simulink model "pfc_desktop"  (R2024b)
settings: configuration reference "CONFI" (kept outside this file)
InitFcn:
  | fidelity_pfc_vals;
  | Fc=66e3;
values from neighbouring files (symbols this model uses):
  Gs = 2e-2    (= 0.02)    [fidelity_pfc_vals.m]
  s = 1    [fidelity_pfc_vals.m]
  stateSpaceParameters_1 =     [stateSpaceParameters.mat]
  t_ss = tsw/30    (= 5.12820512821e-07)    [fidelity_pfc_vals.m]
  tsw = 1/(fsw*1e3)    (= 1.53846153846e-05)    [fidelity_pfc_vals.m]
undefined symbols (not defined in the file or in its folder): a, b, c, DiscIntNeverNeededParam, Down, Up
libraries: fl_lib x40, nesl_utility x37, ee_lib x11, hdlsllib x7, dspsrcs4 x6, eePwmGenerator x3, hdlssclib x2, spsTriangleGeneratorLib x1, simulink x1
(part 3 of 3)

== system pfc_desktop/simscape_system/3Bridges/Simscape/Subsystem5 ==
  g : Inport
  "MOSFET (Ideal, Switching)" : ee_lib/Semiconductors & Converters/MOSFET (Ideal, Switching)  port_option=ee.enum.controlport.ps  Rds=0.01 Ohm  Goff=1e-6 1/Ohm  Vth=2 V  diode_param=ee.enum.semiconductors.protectionDiode.nodynamics  diode_Vf=0.8 V  diode_Ron=0.001 Ohm  diode_Goff=1e-5 1/Ohm  diode_C=50e-9 F  diode_iRM=-235 A  diode_iF=300 A  diode_idot=-50 A/us  diode_trr_param=ee.enum.converters.diodeReverseParam.trr_factor  diode_trr_factor=3  diode_trr=15 us  diode_Qrr=1500 s*uA  ids_specify=off  ids_priority=None  ids=0 A  ids_nominal_specify=off  ids_nominal_value=1  ids_nominal_unit=A  vds_specify=off  vds_priority=None  vds=0 V  vds_nominal_specify=off  vds_nominal_value=1  vds_nominal_unit=V  vgs_specify=off  vgs_priority=None  vgs=0 V  vgs_nominal_specify=off  vgs_nominal_value=1  vgs_nominal_unit=V  thermal_loss_option=ee.enum.converters.thermalLossOption.constantvalues  Von_data=[0, 1.8, 3.2, 6, 10, 16; 0, 2, 5.5, 9.5, 15, 25] V  Tj=[298.15, 448.15] K  Iout_data=[0, 20, 40, 60, 80, 100] A  Eon_data=[0, 55.04, 124.57, 235.53, 362.12; 0, 71.25, 161.25, 304.88, 468.75] * 1e-6 J  Eoff_data=[0, 18, 30, 56.1, 76.5; 0, 22.5, 37.5, 70.13, 95.63] * 1e-6 J  Eon_data_3D=[zeros(2, 5, 3)] J  Eoff_data_3D=[zeros(2, 5, 3)] J  Tj_loss=[298.15, 448.15] K  Iout_data_loss=[0, 10, 20, 30, 40] A  tabulateWithVds=false  Vds_loss=[0, 150, 300] V  Eon_scalar=22.86e-3 J  Eoff_scalar=17.14e-3 J  Voff=300 V  Iout_scalar=600 A  useCurrentFromPreviousCycle=false  useVoltageFromPreviousCycle=false  diodeModelType=ee.enum.converters.diodeModelType.pwl  diodeTableType=ee.enum.diode.tableType.IfMat  diode_ReverseIVType=ee.enum.diode.diodeReverseIV.constant  diode_IfMat=[.07, .12, .19, 1.75, 4.24, 7.32, 11.2; .16, .3, .72, 2.14, 4.02, 6.35, 9.12] A  diode_VfMat=[.9, 1.15, 1.25, 1.5, 1.75, 2.17, 2.6, 2.85; .58, .68, .75, 1.1, 1.38, 1.77, 2.27, 2.7] V  diode_TjVec=[25, 125] degC  diode_VfVec=[.5, .7, .9, 1.3, 1.7, 2.1, 2.5] V  diode_IfVec=[.1, .2, .5, 1, 2, 4, 7, 10] A  diode_IrMat=[1e-06, 2e-06, 5e-06, 1e-05, 2.5e-05, 5e-05, .0001; 2e-06, 5e-06, 1e-05, 4e-05, 8e-05, .0002, .0005] A  diode_VrMat=[10, 100, 200, 250, 300, 325, 350; 10, 70, 160, 220, 270, 300, 320] V  diode_VrVec=[10, 20, 40, 50, 70, 80, 100] V  diode_IrVec=[1e-06, 2e-06, 5e-06, 1e-05, 2e-05, 5e-05, .0001] A  diode_Vr=-600 V  diode_Ls=150 nH  diode_Erec=0.03 J  diode_rec_loss_model=ee.enum.diode.reverseRecoveryModel.fixed  diode_ErecVal=0 J  diode_scaleWithIandV=true  diode_ErecMat=zeros(2, 3) J  diode_TjrecVec=[298.15, 398.15] K  diode_IfrecVec=[.1, 1, 10] A  diode_IrecVal=10 A  diode_VrecVal=10 V  diode_tFilter=1 / 1000 / 100 s  separateThermalPortForDiode=false  thermal_network_parameterization=ee.enum.thermalNetworkTopology.external  Rth=[.03, .2] K/W  Rth_Cauer=[.03, .1, .2] K/W  Rth_Foster=[.08, .14, .22, .16] K/W  thermal_mass_parameterization=ee.enum.thermalNetwork.timeconstant  thermal_mass=[3, 25] J/K  thermal_mass_Cauer=[3, 10, 25] J/K  thermal_mass_Foster=[.001, .005, .05, .5] J/K  thermal_time_constant=[.1, 5] s  thermal_time_constant_Cauer=[.1, 1, 5] s  thermal_time_constant_Foster=[7e-05, .0007, .01, .08] s  thermal_mass_initial_temperatures=[25, 25] degC  thermal_mass_initial_temperatures_Cauer=[25, 25, 25] degC  junction_thermal_mass=0.1 J/K  Tvec_initial_Foster=[25, 25, 25, 25] degC  RthDiode=[.03, .2] K/W  RthCauerDiode=[.03, .1, .2] K/W  RthFosterDiode=[.03, .2] K/W  thermalMassDiode=[3, 25] J/K  thermalMassCauerDiode=[3, 10, 25] J/K  thermalMassFosterDiode=[33, 50] J/K  thermalTauDiode=[.1, 5] s  thermalTauCauerDiode=[.1, 1, 5] s  thermalTauFosterDiode=[1, 10] s  thermalMassInitTempDiode=[25, 25] degC  thermalMassInitTempCauerDiode=[25, 25, 25] degC  junctionthermalMassDiode=0.1 J/K  TVecInitialFosterDiode=[25, 25, 25, 25] degC  no_thermal_network=0  mosfet_junction_temperature_specify=off  mosfet_junction_temperature_priority=None  mosfet_junction_temperature=25 degC  mosfet_junction_temperature_nominal_specify=off  mosfet_junction_temperature_nominal_value=1  mosfet_junction_temperature_nominal_unit=degC  diode_junction_temperature_specify=off  diode_junction_temperature_priority=None  diode_junction_temperature=25 degC  diode_junction_temperature_nominal_specify=off  diode_junction_temperature_nominal_value=1  diode_junction_temperature_nominal_unit=degC  Qj_specify=off  Qj_priority=None  Qj=0 W  Qj_nominal_specify=off  Qj_nominal_value=1  Qj_nominal_unit=W  accumulatedSwitchingLosses_specify=off  accumulatedSwitchingLosses_priority=None  accumulatedSwitchingLosses=0 J
  Simulink-PS Converter : nesl_utility/Simulink-PS Converter  PhysicalDomain=network_engine_domain  SubClassName=ps_input  LeftPortType=input  RightPortType=output  PseudoPeriodic=off  Frequencies=[]  NoiseDistribution=none  NoiseParameters=[]  Unit=1  AffineConversion=off  FilteringAndDerivatives=provide  SimscapeFilterOrder=1  InputFilterTimeConstant=0.001  UdotUserProvided=0
  d : PMIOPort  Side=Left
  s : PMIOPort  Port=2  Side=Right
  wires:
  g/1 -> Simulink-PS Converter/1
  connections:
  "MOSFET (Ideal, Switching)"/RConn1 -- d/RConn1
  "MOSFET (Ideal, Switching)"/RConn2 -- s/RConn1
  Simulink-PS Converter/RConn1 -- "MOSFET (Ideal, Switching)"/LConn1

== system pfc_desktop/simscape_system1/HDL Subsystem/HDL Algorithm/Output ==
  In1 : Inport
  State : Inport  Port=2
  Sel : Inport  Port=3  LockScale=on
  Bias : Terminator
  Mux : Mux  Inputs=2
  Output Update : hdlssclib/NFPSparseConstMultiply  MatrixSource=Dialog  constMatrix=single([stateSpaceParameters_1.Cd stateSpaceParameters_1.Dd])  MatrixType=single  MatrixSize=[1 1]  ColumnIndices=[1]  RowIndices=[1]  PropDataType=single  defWL=48
  Out1 : Outport  VectorParamsAs1DForOutWhenUnconnected=off
  wires:
  State/1 -> Mux/1
  Mux/1 -> Output Update/1
  In1/1 -> Mux/2
  Sel/1 -> Bias/1, Output Update/2
  Output Update/1 -> Out1/1

== system pfc_desktop/simscape_system1/HDL Subsystem/HDL Algorithm/State Update ==
  In1 : Inport
  State : Inport  Port=2
  Sel : Inport  Port=3  LockScale=on
  Bias : Terminator
  Mux : Mux  Inputs=2
  State Update : hdlssclib/NFPSparseConstMultiply  MatrixSource=Dialog  constMatrix=single([stateSpaceParameters_1.Ad stateSpaceParameters_1.Bd])  MatrixType=single  MatrixSize=[1 1]  ColumnIndices=[1]  RowIndices=[1]  PropDataType=single  defWL=43
  State Out : Outport  VectorParamsAs1DForOutWhenUnconnected=off
  wires:
  State/1 -> Mux/1
  In1/1 -> Mux/2
  Mux/1 -> State Update/1
  Sel/1 -> Bias/1, State Update/2
  State Update/1 -> State Out/1

== system pfc_desktop/simscape_system/3Bridges/Linear_FET/MOSFET/Controller ==
  vs : Inport
  is : Inport  Port=2
  G : Inport  Port=3
  Constant : Constant  Value=-.7  SampleTime=-1
  Discrete-Time Integrator : DiscreteIntegrator  IntegratorMethod=Accumulation: Forward Euler  gainval=1/s  SampleTime=-1  OutDataTypeStr=Inherit: Inherit via back propagation  ICPrevOutput=DiscIntNeverNeededParam  ICPrevScaledInput=DiscIntNeverNeededParam
  Equal : RelationalOperator  OutDataTypeStr=boolean  RndMeth=Simplest  InputSameDT=off
  Gain : Gain  Gain=10
  Gain3 : Gain  Gain=Gs  OutDataTypeStr=Inherit: Inherit via back propagation
  Multiply-Add : hdlsllib/HDL Operations/Multiply-Add  Function=c+(a.*b)  datatype=Inherit: Inherit via internal rule  DoSatur=off  FMA=off
  OR : Logic  Operator=OR  IconShape=distinctive  AllPortsSameDT=off  OutDataTypeStr=boolean
  Subtract : Sum  Inputs=+-
  Subtract1 : Sum  Inputs=+-
  Unary Minus : UnaryMinus
  ic : Outport
  wires:
  Multiply-Add/1 -> Subtract/1
  G/1 -> OR/1
  Unary Minus/1 -> Subtract1/1  "on"
  is/1 -> Unary Minus/1
  Discrete-Time Integrator/1 -> ic/1, Subtract/2  "ic"
  Subtract/1 -> Discrete-Time Integrator/1
  vs/1 -> Equal/2, Gain3/1
  Equal/1 -> Gain/1
  Gain/1 -> OR/2
  Constant/1 -> Equal/1
  Gain3/1 -> Subtract1/2, Multiply-Add/3
  Subtract1/1 -> Multiply-Add/1
  OR/1 -> Multiply-Add/2

== system pfc_desktop/simscape_system/3Bridges/Linear_FET/MOSFET1/Controller ==
  vs : Inport
  is : Inport  Port=2
  G : Inport  Port=3
  Constant : Constant  Value=-.7  SampleTime=-1
  Discrete-Time Integrator : DiscreteIntegrator  IntegratorMethod=Accumulation: Forward Euler  gainval=1/s  SampleTime=-1  OutDataTypeStr=Inherit: Inherit via back propagation  ICPrevOutput=DiscIntNeverNeededParam  ICPrevScaledInput=DiscIntNeverNeededParam
  Equal : RelationalOperator  OutDataTypeStr=boolean  RndMeth=Simplest  InputSameDT=off
  Gain : Gain  Gain=10
  Gain3 : Gain  Gain=Gs  OutDataTypeStr=Inherit: Inherit via back propagation
  Multiply-Add : hdlsllib/HDL Operations/Multiply-Add  Function=c+(a.*b)  datatype=Inherit: Inherit via internal rule  DoSatur=off  FMA=off
  OR : Logic  Operator=OR  IconShape=distinctive  AllPortsSameDT=off  OutDataTypeStr=boolean
  Subtract : Sum  Inputs=+-
  Subtract1 : Sum  Inputs=+-
  Unary Minus : UnaryMinus
  ic : Outport
  wires:
  OR/1 -> Multiply-Add/2
  Subtract1/1 -> Multiply-Add/1
  Gain3/1 -> Multiply-Add/3, Subtract1/2
  Constant/1 -> Equal/1
  Gain/1 -> OR/2
  Equal/1 -> Gain/1
  vs/1 -> Gain3/1, Equal/2
  Subtract/1 -> Discrete-Time Integrator/1
  Discrete-Time Integrator/1 -> Subtract/2, ic/1  "ic"
  is/1 -> Unary Minus/1
  Unary Minus/1 -> Subtract1/1  "on"
  G/1 -> OR/1
  Multiply-Add/1 -> Subtract/1

== system pfc_desktop/simscape_system/3Bridges/Linear_FET/MOSFET2/Controller ==
  vs : Inport
  is : Inport  Port=2
  G : Inport  Port=3
  Constant : Constant  Value=-.7  SampleTime=-1
  Discrete-Time Integrator : DiscreteIntegrator  IntegratorMethod=Accumulation: Forward Euler  gainval=1/s  SampleTime=-1  OutDataTypeStr=Inherit: Inherit via back propagation  ICPrevOutput=DiscIntNeverNeededParam  ICPrevScaledInput=DiscIntNeverNeededParam
  Equal : RelationalOperator  OutDataTypeStr=boolean  RndMeth=Simplest  InputSameDT=off
  Gain : Gain  Gain=10
  Gain3 : Gain  Gain=Gs  OutDataTypeStr=Inherit: Inherit via back propagation
  Multiply-Add : hdlsllib/HDL Operations/Multiply-Add  Function=c+(a.*b)  datatype=Inherit: Inherit via internal rule  DoSatur=off  FMA=off
  OR : Logic  Operator=OR  IconShape=distinctive  AllPortsSameDT=off  OutDataTypeStr=boolean
  Subtract : Sum  Inputs=+-
  Subtract1 : Sum  Inputs=+-
  Unary Minus : UnaryMinus
  ic : Outport
  wires:
  Multiply-Add/1 -> Subtract/1
  G/1 -> OR/1
  Unary Minus/1 -> Subtract1/1  "on"
  is/1 -> Unary Minus/1
  Discrete-Time Integrator/1 -> ic/1, Subtract/2  "ic"
  Subtract/1 -> Discrete-Time Integrator/1
  vs/1 -> Equal/2, Gain3/1
  Equal/1 -> Gain/1
  Gain/1 -> OR/2
  Constant/1 -> Equal/1
  Gain3/1 -> Subtract1/2, Multiply-Add/3
  Subtract1/1 -> Multiply-Add/1
  OR/1 -> Multiply-Add/2

== system pfc_desktop/simscape_system/3Bridges/Linear_FET/MOSFET3/Controller ==
  vs : Inport
  is : Inport  Port=2
  G : Inport  Port=3
  Constant : Constant  Value=-.7  SampleTime=-1
  Discrete-Time Integrator : DiscreteIntegrator  IntegratorMethod=Accumulation: Forward Euler  gainval=1/s  SampleTime=-1  OutDataTypeStr=Inherit: Inherit via back propagation  ICPrevOutput=DiscIntNeverNeededParam  ICPrevScaledInput=DiscIntNeverNeededParam
  Equal : RelationalOperator  OutDataTypeStr=boolean  RndMeth=Simplest  InputSameDT=off
  Gain : Gain  Gain=10
  Gain3 : Gain  Gain=Gs  OutDataTypeStr=Inherit: Inherit via back propagation
  Multiply-Add : hdlsllib/HDL Operations/Multiply-Add  Function=c+(a.*b)  datatype=Inherit: Inherit via internal rule  DoSatur=off  FMA=off
  OR : Logic  Operator=OR  IconShape=distinctive  AllPortsSameDT=off  OutDataTypeStr=boolean
  Subtract : Sum  Inputs=+-
  Subtract1 : Sum  Inputs=+-
  Unary Minus : UnaryMinus
  ic : Outport
  wires:
  OR/1 -> Multiply-Add/2
  Subtract1/1 -> Multiply-Add/1
  Gain3/1 -> Multiply-Add/3, Subtract1/2
  Constant/1 -> Equal/1
  Gain/1 -> OR/2
  Equal/1 -> Gain/1
  vs/1 -> Gain3/1, Equal/2
  Subtract/1 -> Discrete-Time Integrator/1
  Discrete-Time Integrator/1 -> Subtract/2, ic/1  "ic"
  is/1 -> Unary Minus/1
  Unary Minus/1 -> Subtract1/1  "on"
  G/1 -> OR/1
  Multiply-Add/1 -> Subtract/1

== system pfc_desktop/simscape_system/3Bridges/Linear_FET/MOSFET4/Controller ==
  vs : Inport
  is : Inport  Port=2
  G : Inport  Port=3
  Constant : Constant  Value=-.7  SampleTime=-1
  Discrete-Time Integrator : DiscreteIntegrator  IntegratorMethod=Accumulation: Forward Euler  gainval=1/s  SampleTime=-1  OutDataTypeStr=Inherit: Inherit via back propagation  ICPrevOutput=DiscIntNeverNeededParam  ICPrevScaledInput=DiscIntNeverNeededParam
  Equal : RelationalOperator  OutDataTypeStr=boolean  RndMeth=Simplest  InputSameDT=off
  Gain : Gain  Gain=10
  Gain3 : Gain  Gain=Gs  OutDataTypeStr=Inherit: Inherit via back propagation
  Multiply-Add : hdlsllib/HDL Operations/Multiply-Add  Function=c+(a.*b)  datatype=Inherit: Inherit via internal rule  DoSatur=off  FMA=off
  OR : Logic  Operator=OR  IconShape=distinctive  AllPortsSameDT=off  OutDataTypeStr=boolean
  Subtract : Sum  Inputs=+-
  Subtract1 : Sum  Inputs=+-
  Unary Minus : UnaryMinus
  ic : Outport
  wires:
  Multiply-Add/1 -> Subtract/1
  G/1 -> OR/1
  Unary Minus/1 -> Subtract1/1  "on"
  is/1 -> Unary Minus/1
  Discrete-Time Integrator/1 -> ic/1, Subtract/2  "ic"
  Subtract/1 -> Discrete-Time Integrator/1
  vs/1 -> Equal/2, Gain3/1
  Equal/1 -> Gain/1
  Gain/1 -> OR/2
  Constant/1 -> Equal/1
  Gain3/1 -> Subtract1/2, Multiply-Add/3
  Subtract1/1 -> Multiply-Add/1
  OR/1 -> Multiply-Add/2

== system pfc_desktop/simscape_system/3Bridges/Linear_FET/MOSFET5/Controller ==
  vs : Inport
  is : Inport  Port=2
  G : Inport  Port=3
  Constant : Constant  Value=-.7  SampleTime=-1
  Discrete-Time Integrator : DiscreteIntegrator  IntegratorMethod=Accumulation: Forward Euler  gainval=1/s  SampleTime=-1  OutDataTypeStr=Inherit: Inherit via back propagation  ICPrevOutput=DiscIntNeverNeededParam  ICPrevScaledInput=DiscIntNeverNeededParam
  Equal : RelationalOperator  OutDataTypeStr=boolean  RndMeth=Simplest  InputSameDT=off
  Gain : Gain  Gain=10
  Gain3 : Gain  Gain=Gs  OutDataTypeStr=Inherit: Inherit via back propagation
  Multiply-Add : hdlsllib/HDL Operations/Multiply-Add  Function=c+(a.*b)  datatype=Inherit: Inherit via internal rule  DoSatur=off  FMA=off
  OR : Logic  Operator=OR  IconShape=distinctive  AllPortsSameDT=off  OutDataTypeStr=boolean
  Subtract : Sum  Inputs=+-
  Subtract1 : Sum  Inputs=+-
  Unary Minus : UnaryMinus
  ic : Outport
  wires:
  OR/1 -> Multiply-Add/2
  Subtract1/1 -> Multiply-Add/1
  Gain3/1 -> Multiply-Add/3, Subtract1/2
  Constant/1 -> Equal/1
  Gain/1 -> OR/2
  Equal/1 -> Gain/1
  vs/1 -> Gain3/1, Equal/2
  Subtract/1 -> Discrete-Time Integrator/1
  Discrete-Time Integrator/1 -> Subtract/2, ic/1  "ic"
  is/1 -> Unary Minus/1
  Unary Minus/1 -> Subtract1/1  "on"
  G/1 -> OR/1
  Multiply-Add/1 -> Subtract/1

== stateflow chart pfc_desktop/control/Function-call scheduler ==
  state Run
    send(xFunction);
  (default) -> Run
  events: xFunction output FUNCTION_CALL_EVENT
